simulink subsystem "MOTOR"  (R2024a)
settings: Solver=VariableStepAuto  StartTime=0.0  StopTime=10.0  RelTol=1e-3
undefined symbols (not defined in the file): b, J, K, L, R
settings Model: Creator=nacer  LastModifiedBy=nacer

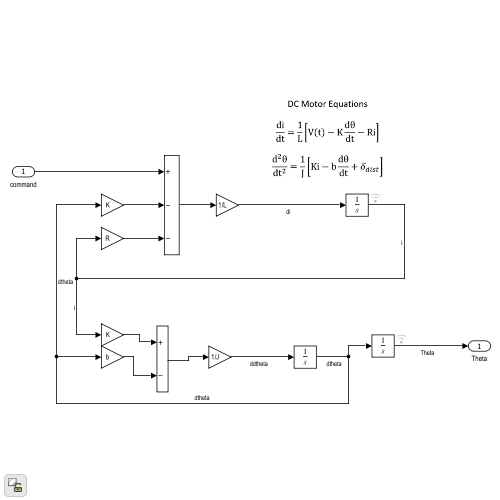
[thumbnail: Simulink's stored preview of the top-level diagram]
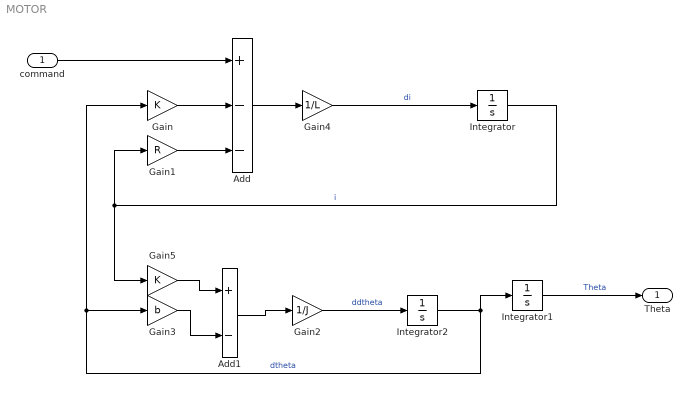
== system MOTOR ==
  command : Inport
  Add : Sum  Inputs=+--
  Add1 : Sum  Inputs=+-
  Gain : Gain  Gain=K
  Gain1 : Gain  Gain=R
  Gain2 : Gain  Gain=1/J
  Gain3 : Gain  Gain=b
  Gain4 : Gain  Gain=1/L
  Gain5 : Gain  Gain=K
  Integrator : Integrator
  Integrator1 : Integrator
  Integrator2 : Integrator
  Theta : Outport
  wires:
  Gain/1 -> Add/2
  Integrator/1 -> Gain5/1, Gain1/1  "i"
  Gain3/1 -> Add1/2
  Gain4/1 -> Integrator/1  "di"
  Gain5/1 -> Add1/1
  Add/1 -> Gain4/1
  Gain1/1 -> Add/3
  Add1/1 -> Gain2/1
  Gain2/1 -> Integrator2/1  "ddtheta"
  Integrator2/1 -> Gain/1, Gain3/1, Integrator1/1  "dtheta"
  Integrator1/1 -> Theta/1  "Theta"
  command/1 -> Add/1
